simulink model "observersimualtion"  (R2017a)
settings: Solver=ode45  StartTime=0.0  StopTime=20  RelTol=1e-6  EnableMultiTasking=on
values from neighbouring files (symbols this model uses):
  d0 = 1.5897e-3    (= 0.0015897)    [init_paramters.m]
  d1 = 1.773e-6    (= 1.773e-06)    [init_paramters.m]
  g = 9.81    [init_paramters.m]
  J0 = 1.4316e-4    (= 0.00014316)    [init_paramters.m]
  J1 = 2.078867e-4    (= 0.0002078867)    [init_paramters.m]
  Kf = 0.05722    [init_paramters.m]
  Kg = 13/18    (= 0.722222222222)    [init_paramters.m]
  Kt = 0.05722    [init_paramters.m]
  L0 = 0.09    [init_paramters.m]
  L1 = 0.225    [init_paramters.m]
  m1 = 0.009    [init_paramters.m]
  Ra = 17    [init_paramters.m]
libraries: sharedTrackingLibrary x1
settings Model: Creator=Alvin  LastModifiedBy=alvin
settings SolverCC: AlgebraicLoopSolver=LineSearch
settings DataIOCC: LimitDataPoints=on  SaveFormat=Array  SaveState=on
settings OptimizationCC: LifeSpan=inf
settings DebuggingCC: SFUnexpectedBacktrackingDiag=warning  SFNoUnconditionalDefaultTransitionDiag=warning  SFExecutionAtInitializationDiag=none
settings HardwareCC: ProdBitPerPointer=32  ProdBitPerSizeT=32  ProdBitPerPtrDiffT=32  ProdLargestAtomicFloat=None  ProdIntDivRoundTo=Undefined  ProdEndianess=Unspecified  ProdWordSize=32  ProdHWDeviceType=32-bit Generic
settings ModelReferenceCC: PropagateSignalLabelsOutOfModel=off
settings GRTTargetCC: TargetLangStandard=C89/C90 (ANSI)  GeneratePreprocessorConditionals=Disable all
settings ConfigComp: CovMetricSettings=dw  CovHtmlReporting=on  CovSaveCumulativeToWorkspaceVar=on  CovSaveSingleToWorkspaceVar=on  CovExternalEMLEnable=off

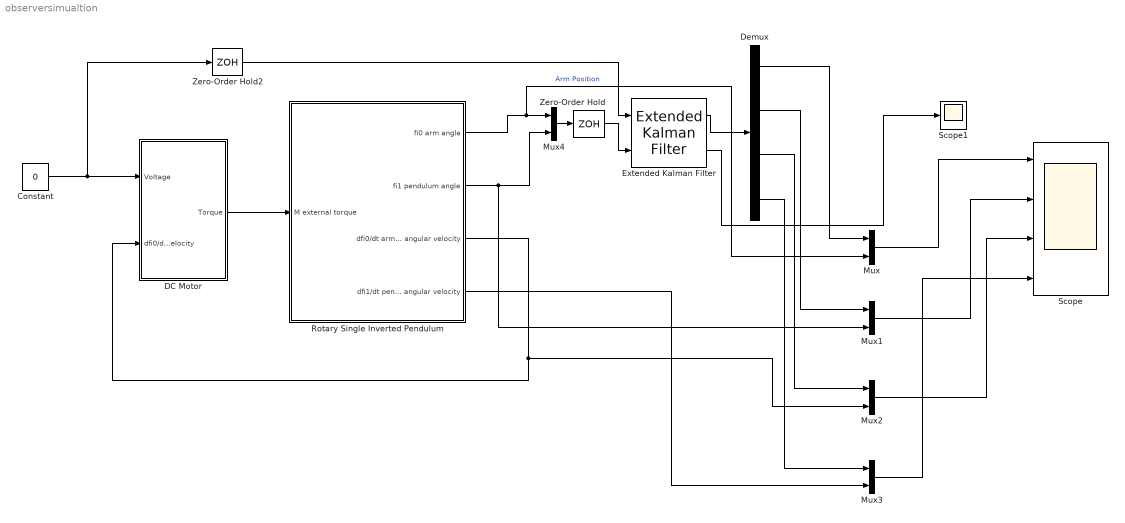
== system observersimualtion ==
  Constant : Constant  Value=0
  DC Motor : Subsystem
  Demux : Demux
  Extended Kalman Filter : sharedTrackingLibrary/Extended Kalman Filter  StateTransitionFcn=myStateTransitionFcn  HasStateTransitionJacobianFcn=off  HasAdditiveProcessNoise=Additive  ProcessNoise=diag([1 1 0 0])  HasTimeVaryingProcessNoise=off  HasStateTransitionFcnExtraArgument=1  InitialState=[0 5.0 0 0]  InitialStateCovariance=0.001  MeasurementFcn1=myMeasurementFcn  HasMeasurementJacobianFcn1=off  HasMeasurementEnablePort1=off  HasAdditiveMeasurementNoise1=Additive  MeasurementNoise1=[1;1]  HasTimeVaryingMeasurementNoise1=off  HasMeasurementFcnExtraArgument1=0  MeasurementFcn2=myMeasurementFcn  HasMeasurementJacobianFcn2=off  HasMeasurementEnablePort2=off  HasAdditiveMeasurementNoise2=Additive  MeasurementNoise2=1  HasTimeVaryingMeasurementNoise2=off  HasMeasurementFcnExtraArgument2=0  MeasurementFcn3=myMeasurementFcn  HasMeasurementJacobianFcn3=off  HasMeasurementEnablePort3=off  HasAdditiveMeasurementNoise3=Additive  MeasurementNoise3=1  HasTimeVaryingMeasurementNoise3=off  HasMeasurementFcnExtraArgument3=0  MeasurementFcn4=myMeasurementFcn  HasMeasurementJacobianFcn4=off  HasMeasurementEnablePort4=off  HasAdditiveMeasurementNoise4=Additive  MeasurementNoise4=1  HasTimeVaryingMeasurementNoise4=off  HasMeasurementFcnExtraArgument4=0  MeasurementFcn5=myMeasurementFcn  HasMeasurementJacobianFcn5=off  HasMeasurementEnablePort5=off  HasAdditiveMeasurementNoise5=Additive  MeasurementNoise5=1  HasTimeVaryingMeasurementNoise5=off  HasMeasurementFcnExtraArgument5=0  EnableMultirate=off  StateTransitionFcnSampleTime=1  MeasurementFcn1SampleTime=1  MeasurementFcn2SampleTime=1  MeasurementFcn3SampleTime=1  MeasurementFcn4SampleTime=1  MeasurementFcn5SampleTime=1  UseCurrentEstimator=on  OutputStateCovariance=on  DataType=double  SampleTime=0.025  NumberOfMeasurements=1
  Mux{,1..4} (5 alike) : Mux  Inputs=2
  Rotary Single Inverted Pendulum : Subsystem  mask{fi1=5.0}
      mask prompts: fi1 "Pendulum Position Initial Condition"
      mask TypeOptions fi1: Pendulum/Constant/Value
  Scope : Scope  NumInputPorts=4
  Scope1 : Scope
  Zero-Order Hold : ZeroOrderHold  SampleTime=0.025
  Zero-Order Hold2 : ZeroOrderHold  SampleTime=0.025
  wires:
  DC Motor/1(Torque) -> Rotary Single Inverted Pendulum/1(M external torque)
  Constant/1 -> Zero-Order Hold2/1, DC Motor/1(Voltage)
  Zero-Order Hold2/1 -> Extended Kalman Filter/1
  Extended Kalman Filter/1 -> Demux/1
  Demux/1 -> Mux/1
  Demux/2 -> Mux1/1
  Demux/3 -> Mux2/1
  Demux/4 -> Mux3/1
  Mux/1 -> Scope/1
  Mux1/1 -> Scope/2
  Mux2/1 -> Scope/3
  Mux3/1 -> Scope/4
  Rotary Single Inverted Pendulum/3(dfi0/dt arm angular velocity) -> Mux2/2, DC Motor/2(dfi0/dt Arm Angular Velocity)
  Rotary Single Inverted Pendulum/4(dfi1/dt pendulum angular velocity) -> Mux3/2
  Rotary Single Inverted Pendulum/1(fi0 arm angle) -> Mux/2, Mux4/1  "Arm Position"
  Rotary Single Inverted Pendulum/2(fi1 pendulum angle) -> Mux1/2, Mux4/2
  Mux4/1 -> Zero-Order Hold/1
  Zero-Order Hold/1 -> Extended Kalman Filter/2
  Extended Kalman Filter/2 -> Scope1/1

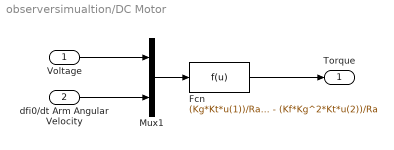
== system observersimualtion/DC Motor ==
  Voltage : Inport
  dfi0/dt Arm Angular Velocity : Inport  Port=2
  Fcn : Fcn  Expr=(Kg*Kt*u(1))/Ra - (Kf*Kg^2*Kt*u(2))/Ra
  Mux1 : Mux  Inputs=2
  Torque : Outport
  wires:
  dfi0/dt Arm Angular Velocity/1 -> Mux1/2
  Mux1/1 -> Fcn/1
  Fcn/1 -> Torque/1
  Voltage/1 -> Mux1/1

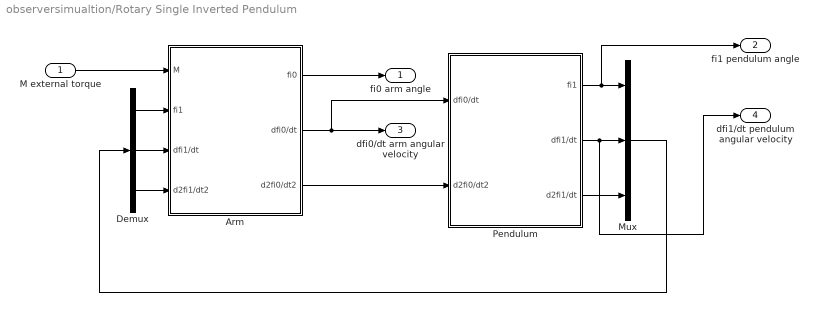
== system observersimualtion/Rotary Single Inverted Pendulum ==
  M external torque : Inport
  Arm : Subsystem
  Demux : Demux  Outputs=3
  Mux : Mux  Inputs=3
  Pendulum : Subsystem
  fi0 arm angle : Outport
  fi1 pendulum angle : Outport  Port=2
  dfi0/dt arm angular velocity : Outport  Port=3
  dfi1/dt pendulum angular velocity : Outport  Port=4
  wires:
  Pendulum/1(fi1) -> fi1 pendulum angle/1, Mux/1
  Pendulum/2(dfi1/dt) -> dfi1/dt pendulum angular velocity/1, Mux/2
  Mux/1 -> Demux/1
  Demux/1 -> Arm/2(fi1)
  Demux/2 -> Arm/3(dfi1/dt)
  Demux/3 -> Arm/4(d2fi1/dt2)
  M external torque/1 -> Arm/1(M)
  Pendulum/3(d2fi1/dt) -> Mux/3
  Arm/3(d2fi0/dt2) -> Pendulum/2(d2fi0/dt2)
  Arm/1(fi0) -> fi0 arm angle/1
  Arm/2(dfi0/dt) -> dfi0/dt arm angular velocity/1, Pendulum/1(dfi0/dt)

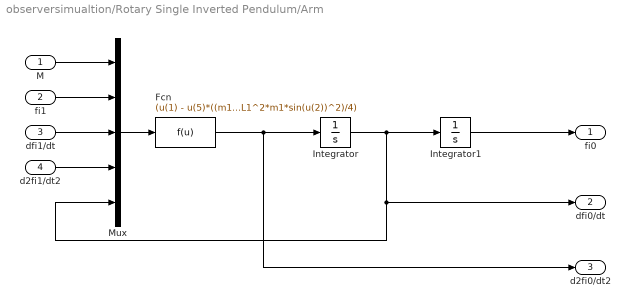
== system observersimualtion/Rotary Single Inverted Pendulum/Arm ==
  M : Inport
  fi1 : Inport  Port=2
  dfi1/dt : Inport  Port=3
  d2fi1/dt2 : Inport  Port=4
  Fcn : Fcn  Expr=(u(1) - u(5)*((m1*u(3)*sin(2*u(2))*L1^2)/4 + d0) + (L0*L1*m1*u(3)^2*sin(u(2)))/2 - (L0*L1*m1*u(4)*cos(u(2)))/2)/(J0 + L0^2*m1 + (L1^2*m1*sin(u(2))^2)/4)
  Integrator : Integrator
  Integrator1 : Integrator
  Mux : Mux  Inputs=5
  fi0 : Outport
  dfi0/dt : Outport  Port=2
  d2fi0/dt2 : Outport  Port=3
  wires:
  Mux/1 -> Fcn/1
  Fcn/1 -> d2fi0/dt2/1, Integrator/1
  Integrator/1 -> dfi0/dt/1, Mux/5, Integrator1/1
  Integrator1/1 -> fi0/1
  fi1/1 -> Mux/2
  dfi1/dt/1 -> Mux/3
  M/1 -> Mux/1
  d2fi1/dt2/1 -> Mux/4

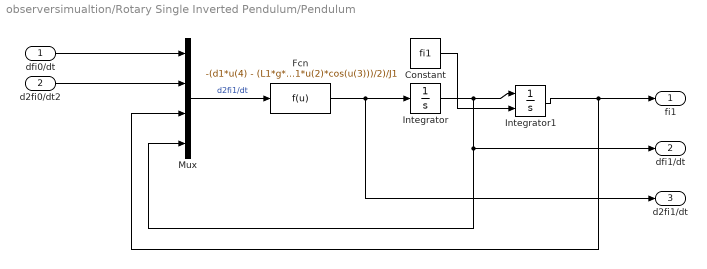
== system observersimualtion/Rotary Single Inverted Pendulum/Pendulum ==
  dfi0/dt : Inport
  d2fi0/dt2 : Inport  Port=2
  Constant : Constant  Value=fi1
  Fcn : Fcn  Expr=-(d1*u(4) - (L1*g*m1*sin(u(3)))/2 - (L1^2*m1*u(1)^2*sin(2*u(3)))/8 + (L0*L1*m1*u(2)*cos(u(3)))/2)/J1
  Integrator : Integrator
  Integrator1 : Integrator  InitialConditionSource=external
  Mux : Mux
  fi1 : Outport
  dfi1/dt : Outport  Port=2
  d2fi1/dt : Outport  Port=3
  wires:
  Integrator1/1 -> fi1/1, Mux/3
  Fcn/1 -> d2fi1/dt/1, Integrator/1
  Mux/1 -> Fcn/1  "d2fi1/dt"
  Integrator/1 -> dfi1/dt/1, Mux/4, Integrator1/1
  dfi0/dt/1 -> Mux/1
  d2fi0/dt2/1 -> Mux/2
  Constant/1 -> Integrator1/2
